simulink model "TClntDspl"  (R2016b)
settings: Solver=VariableStepAuto  StartTime=0.0  StopTime=10.0  RelTol=1e-3
settings Model: Creator=jiakui  LastModifiedBy=jiakui

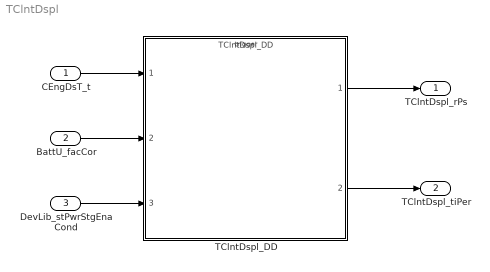
== system TClntDspl ==
  CEngDsT_t : Inport  Tag=deg  Description=engine coolant temperature after filter  OutMin=-200  OutMax=200  OutDataTypeStr=Temp_deg
  BattU_facCor : Inport  Description=Battery correction factor  Port=2  OutMin=-32  OutMax=31.9  OutDataTypeStr=Factor
  DevLib_stPwrStgEnaCond : Inport  Description=Control unit status relevant to power stage deactivation/error diagnosis  Port=3  OutMin=0  OutMax=65535  OutDataTypeStr=State_uint16
  TClntDspl_DD : ModelReference  ModelNameDialog=TClntDspl_DD  SimulationMode=Normal  ModelReferenceVersion=1.24  TriggerPortName=function  TriggerPortTriggerType=function-call  TriggerPortStatesWhenEnabling=held
  TClntDspl_rPs : Outport  Tag=%  Description=Output to the power stage of coolant temperature PWM output to drive the gauge on the dashboard  OutMin=0  OutMax=100  OutDataTypeStr=DutyCycle_rate
  TClntDspl_tiPer : Outport  Tag=us  Description=Class Instance for PWM / Reference value for period duration (small type to limit dynamic range)  Port=2  OutMin=-107374182  OutMax=107374182  OutDataTypeStr=Time_PwmHigh_us
  wires:
  CEngDsT_t/1 -> TClntDspl_DD/1
  BattU_facCor/1 -> TClntDspl_DD/2
  DevLib_stPwrStgEnaCond/1 -> TClntDspl_DD/3
  TClntDspl_DD/1 -> TClntDspl_rPs/1
  TClntDspl_DD/2 -> TClntDspl_tiPer/1
